simulink model "xpcUEIasync"  (Simulink 6.0)
settings: Solver=FixedStepDiscrete  StartTime=0.0  StopTime=inf  FixedStep=.001  RelTol=1e-3
undefined symbols (not defined in the file or in its folder): MF, PD2
libraries: xpclib x4, dspsigattribs x1
settings Model: Creator=gweast  LastModifiedBy=ekbas  ExtModeArmWhenConnect=off  BufferReuse=off  ProdHWDeviceType=Specified  xpc_rtwmakecfg_data=_xpcuei_
settings DataIOCC: SignalLoggingName=sigsOut
settings OptimizationCC: InlineInvariantSignals=off  OptimizeBlockIOStorage=off  BufferReuse=off  EnforceIntegerDowncast=off  FoldNonRolledExpr=off  LocalBlockOutputs=off  MultiInstanced=off
settings FormatCC: IgnoreBidirectionalLines=off
settings HardwareCC: ProdHWDeviceType=Specified
settings RTWCC: SystemTargetFile=xpctarget.tlc  TemplateMakefile=xpc_default_tmf  ProcessScript=xpctarget_make_rtw_hook
settings CodeAppCC: SimulinkBlockComments=off
settings xpcTargetCC: TargetFcnLib=iso_c_tmw.mat

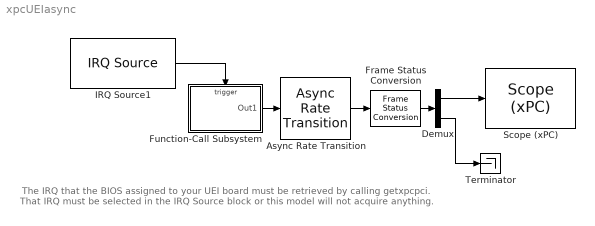
== system xpcUEIasync ==
  note: The IRQ that the BIOS assigned to your UEI board
      | must be retrieved by calling getxpcpci.  That IRQ
      | must be selected in the IRQ Source block or this
      | model will not acquire anything.
  Async Rate Transition : xpclib/Asynchronous Event/Async Rate Transition  sample_time=-1
  Demux : Demux  Outputs=[5 -1]
  Frame Status Conversion : dspsigattribs/Frame Status Conversion  growRefPort=off  outframe=Sample-based
  Function-Call Subsystem : Subsystem  TreatAsAtomicUnit=on
  IRQ Source1 : xpclib/Asynchronous Event/IRQ Source  irqNo=10  preempt=on  b_type=UEI_MFx  slot=-1
  "Scope (xPC) " : xpclib/Misc./Scope (xPC)   scopeno=1  scopetype=Target  autostart=on  viewmode=Graphical redraw  formatstr='%15.6f'  grid=on  ylimits=[0,0]  nosamples=500  noprepostsamples=0  interleave=1  triggermode=FreeRun  triggersignal=1  triggerlevel=0.0  triggerslope=Either  triggerscope=1  triggersample=0  filename=data.dat  mode=Lazy  writesize=512  autorestart=off
  Terminator : Terminator
  wires:
  IRQ Source1/1 -> Function-Call Subsystem/Trigger
  Function-Call Subsystem/1(Out1) -> Async Rate Transition/1
  Frame Status Conversion/1 -> Demux/1
  Demux/1 -> "Scope (xPC) "/1
  Demux/2 -> Terminator/1
  Async Rate Transition/1 -> Frame Status Conversion/1

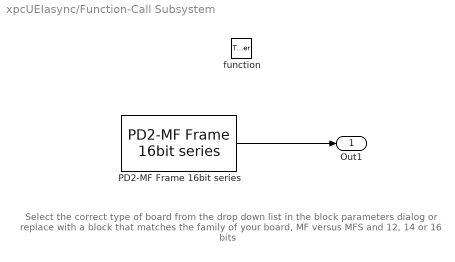
== system xpcUEIasync/Function-Call Subsystem ==
  note: Select the correct type of board from the drop down list
      | in the block parameters dialog or replace with a block
      | that matches the family of your board, MF versus MFS
      | and 12, 14 or 16 bits
  function : TriggerPort  TriggerType=function-call
  "PD2-MF Frame 16bit series " : xpclib/A//D Frame/UEI/PD2-MF Frame 16bit series   boardtypein=PD2-MF-16-333/16H  channel=[1]  gain=[1]  mux=[0]  range=+- 10 Volts  sediff=Single Ended  framesize=32  outfmt=Frame (Signal Processing blockset needed)  clsource=Internal  scantime=-1  frametime=0.001  sampletime=on  slave=off  freq=-1  burst=32  pcislot=-1
  Out1 : Outport
  wires:
  "PD2-MF Frame 16bit series "/1 -> Out1/1
